simulink model "Proj_v3_wF_Transient"  (R2021b)
settings: Solver=FixedStepAuto  StartTime=0.0  StopTime=10000  FixedStep=10  RelTol=1e-3
values from neighbouring files (symbols this model uses):
  b = 0.0007363716    [Proj_v3_1_mat.m]    (also in Proj_v3_mat.m)
  delta = 3.1e-4    (= 0.00031)    [Proj_v3_1_mat.m]    (also in Proj_v3_mat.m)
  F_L = 0.26    [Proj_v3_1_mat.m]    (also in Proj_v3_mat.m)
  F_P = 0.75    [Proj_v3_1_mat.m]    (also in Proj_v3_mat.m)
  k = 0.7931544    [Proj_v3_1_mat.m]    (also in Proj_v3_mat.m)
  K_m = 16.55418    [Proj_v3_1_mat.m]    (also in Proj_v3_mat.m)
  m = 0.75    [Proj_v3_1_mat.m]    (also in Proj_v3_mat.m)
  r = dose/L    (= 233.333333333)    [Proj_v3_1_mat.m]    (also in Proj_v3_mat.m)
  R_A = 0.0705    [Proj_v3_1_mat.m]    (also in Proj_v3_mat.m)
  S = 0    [Proj_v3_1_mat.m]    (also in Proj_v3_mat.m)
  s = 1.5    [Proj_v3_1_mat.m]    (also in Proj_v3_mat.m)
  V_L = (((W*0.0148)*1000)/rho_liver)/1000    (= 1.17876106195)    [Proj_v3_1_mat.m]    (also in Proj_v3_mat.m)
  V_max = 3.0265    [Proj_v3_1_mat.m]    (also in Proj_v3_mat.m)
  V_T = (W/1.01)*(1-0.064-0.12-0.0148)    (= 71.3940594059)    [Proj_v3_1_mat.m]    (also in Proj_v3_mat.m)
  V_v = 0.064*W    (= 5.76)    [Proj_v3_1_mat.m]    (also in Proj_v3_mat.m)
settings Model: Creator=samil  LastModifiedBy=samil

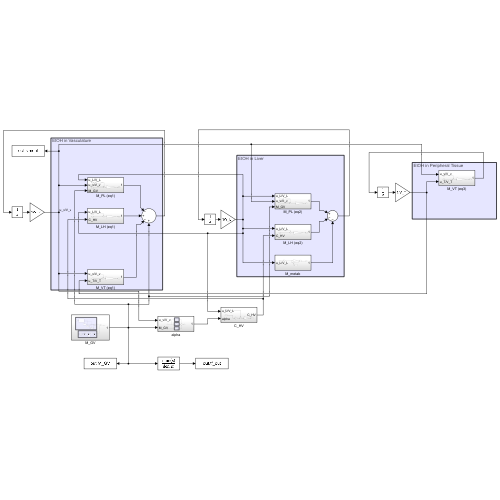
[thumbnail: Simulink's stored preview of the top-level diagram]
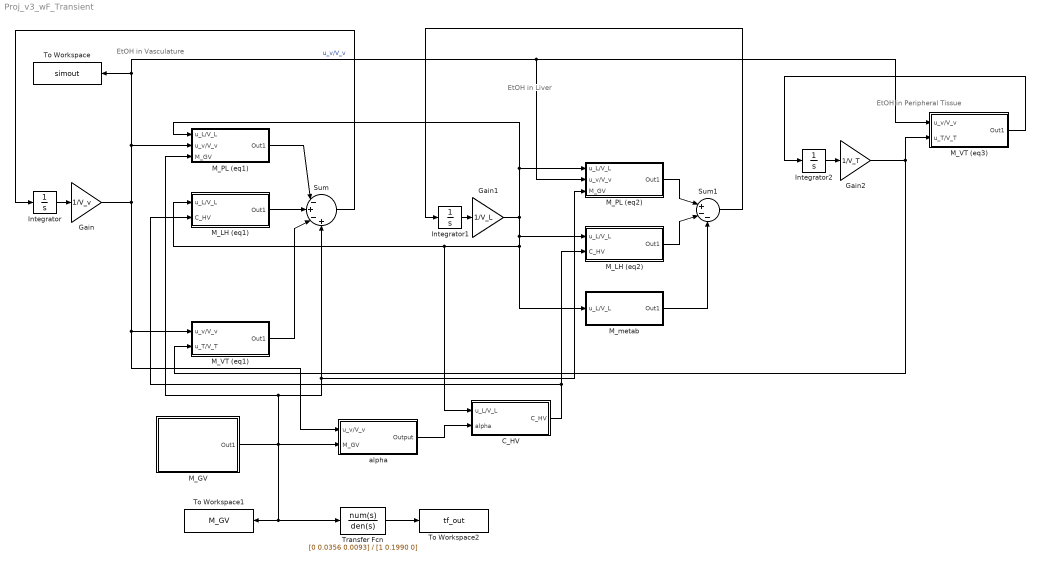
== system Proj_v3_wF_Transient ==
  note: EtOH in Vasculature
  note: EtOH in Peripheral Tissue
  note: EtOH in Liver
  C_HV : Subsystem
  Gain : Gain  Gain=1/V_v
  Gain1 : Gain  Gain=1/V_L
  Gain2 : Gain  Gain=1/V_T
  Integrator : Integrator
  Integrator1 : Integrator
  Integrator2 : Integrator
  M_GV : Subsystem
  M_LH (eq1) : Subsystem
  M_LH (eq2) : Subsystem
  M_PL (eq1) : Subsystem
  M_PL (eq2) : Subsystem
  M_VT (eq1) : Subsystem
  M_VT (eq3) : Subsystem
  M_metab : Subsystem
  Sum : Sum  Inputs=|-+-+
  Sum1 : Sum  Inputs=|+--
  To Workspace : ToWorkspace  VariableName=simout  SaveFormat=Timeseries  SampleTime=-1
  To Workspace1 : ToWorkspace  VariableName=M_GV  SaveFormat=Timeseries  SampleTime=-1
  To Workspace2 : ToWorkspace  VariableName=tf_out  SaveFormat=Timeseries  SampleTime=-1
  Transfer Fcn : TransferFcn  Numerator=[0 0.0356 0.0093]  Denominator=[1 0.1990 0]
  alpha : Subsystem
  wires:
  Integrator1/1 -> Gain1/1
  Integrator2/1 -> Gain2/1
  Integrator/1 -> Gain/1
  Sum/1 -> Integrator/1
  Sum1/1 -> Integrator1/1
  Gain/1 -> To Workspace/1, M_VT (eq3)/1(u_v/V_v), M_PL (eq2)/2(u_v/V_v), M_PL (eq1)/2(u_v/V_v), alpha/1(u_v/V_v), M_VT (eq1)/1(u_v/V_v)  "u_v/V_v"
  C_HV/1(C_HV) -> M_LH (eq1)/2(C_HV), M_LH (eq2)/2(C_HV)
  Gain1/1 -> C_HV/1(u_L/V_L), M_LH (eq1)/1(u_L/V_L), M_metab/1(u_L/V_L), M_LH (eq2)/1(u_L/V_L), M_PL (eq1)/1(u_L/V_L), M_PL (eq2)/1(u_L/V_L)
  Gain2/1 -> M_VT (eq1)/2(u_T/V_T), M_VT (eq3)/2(u_T/V_T)
  alpha/1(Output) -> C_HV/2(alpha)
  M_GV/1(Out1) -> M_PL (eq1)/3(M_GV), Sum/4, M_PL (eq2)/3(M_GV), alpha/2(M_GV), Transfer Fcn/1, To Workspace1/1
  M_PL (eq1)/1(Out1) -> Sum/1
  M_LH (eq1)/1(Out1) -> Sum/2
  M_VT (eq1)/1(Out1) -> Sum/3
  M_PL (eq2)/1(Out1) -> Sum1/1
  M_LH (eq2)/1(Out1) -> Sum1/2
  M_metab/1(Out1) -> Sum1/3
  M_VT (eq3)/1(Out1) -> Integrator2/1
  Transfer Fcn/1 -> To Workspace2/1

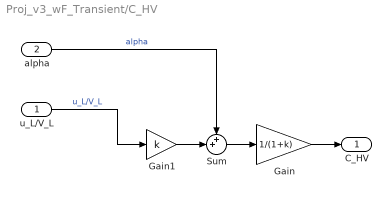
== system Proj_v3_wF_Transient/C_HV ==
  u_L/V_L : Inport
  alpha : Inport  Port=2
  Gain : Gain  Gain=1/(1+k)
  Gain1 : Gain  Gain=k
  Sum : Sum  Inputs=++|
  C_HV : Outport
  wires:
  alpha/1 -> Sum/1  "alpha"
  u_L/V_L/1 -> Gain1/1  "u_L/V_L"
  Gain1/1 -> Sum/2
  Sum/1 -> Gain/1
  Gain/1 -> C_HV/1

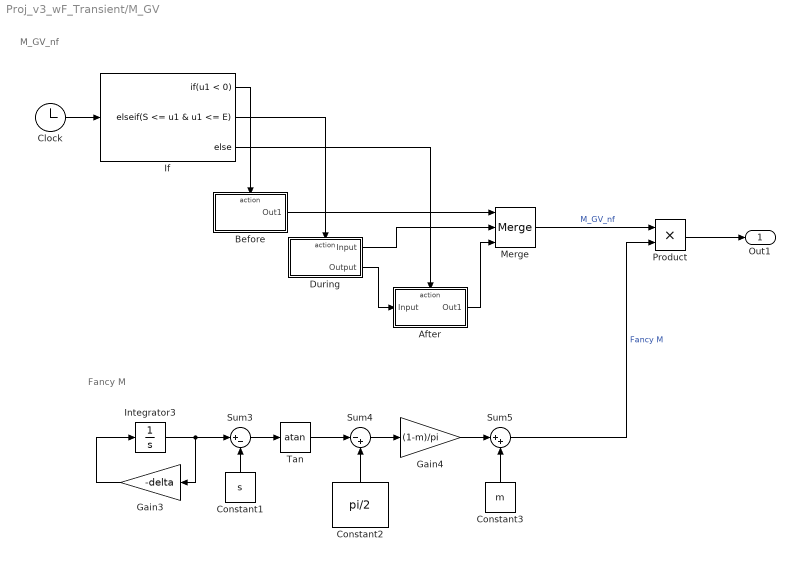
== system Proj_v3_wF_Transient/M_GV ==
  note: Fancy M
  note: M_GV_nf
  After : Subsystem  TreatAsAtomicUnit=on
  Before : Subsystem  TreatAsAtomicUnit=on
  Clock : Clock
  Constant1 : Constant  Value=s
  Constant2 : Constant  Value=pi/2
  Constant3 : Constant  Value=m
  During : Subsystem  TreatAsAtomicUnit=on
  Gain3 : Gain  Gain=-delta
  Gain4 : Gain  Gain=(1-m)/pi
  If : If  IfExpression=u1 < 0  ElseIfExpressions=S <= u1 & u1 <= E
  Integrator3 : Integrator
  Merge : Merge  Inputs=3
  Product : Product
  Sum3 : Sum  Inputs=|+-
  Sum4 : Sum  Inputs=|-+
  Sum5 : Sum  Inputs=|++
  Tan : Trigonometry  Operator=atan
  Out1 : Outport
  wires:
  If/1 -> Before/Action
  If/2 -> During/Action
  Clock/1 -> If/1
  Tan/1 -> Sum4/1
  During/2(Output) -> After/1(Input)
  Product/1 -> Out1/1
  During/1(Input) -> Merge/2
  Integrator3/1 -> Sum3/1, Gain3/1
  If/3 -> After/Action
  Merge/1 -> Product/1  "M_GV_nf"
  Before/1(Out1) -> Merge/1
  Constant3/1 -> Sum5/2
  Sum5/1 -> Product/2  "Fancy M"
  After/1(Out1) -> Merge/3
  Gain4/1 -> Sum5/1
  Sum3/1 -> Tan/1
  Constant1/1 -> Sum3/2
  Constant2/1 -> Sum4/2
  Sum4/1 -> Gain4/1
  Gain3/1 -> Integrator3/1

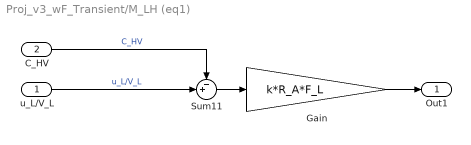
== system Proj_v3_wF_Transient/M_LH (eq1) ==
  u_L/V_L : Inport
  C_HV : Inport  Port=2
  Gain : Gain  Gain=k*R_A*F_L
  Sum11 : Sum  Inputs=-+|
  Out1 : Outport
  wires:
  Sum11/1 -> Gain/1
  u_L/V_L/1 -> Sum11/2  "u_L/V_L"
  C_HV/1 -> Sum11/1  "C_HV"
  Gain/1 -> Out1/1

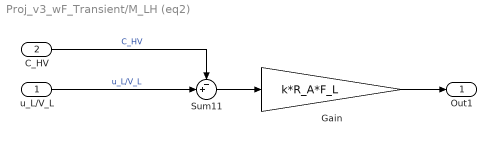
== system Proj_v3_wF_Transient/M_LH (eq2) ==
  u_L/V_L : Inport
  C_HV : Inport  Port=2
  Gain : Gain  Gain=k*R_A*F_L
  Sum11 : Sum  Inputs=-+|
  Out1 : Outport
  wires:
  u_L/V_L/1 -> Sum11/2  "u_L/V_L"
  C_HV/1 -> Sum11/1  "C_HV"
  Sum11/1 -> Gain/1
  Gain/1 -> Out1/1

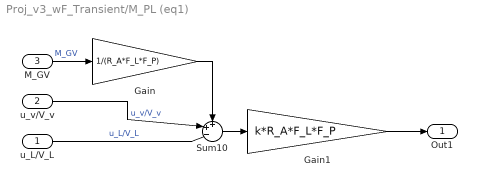
== system Proj_v3_wF_Transient/M_PL (eq1) ==
  u_L/V_L : Inport
  u_v/V_v : Inport  Port=2
  M_GV : Inport  Port=3
  Gain : Gain  Gain=1/(R_A*F_L*F_P)
  Gain1 : Gain  Gain=k*R_A*F_L*F_P
  Sum10 : Sum  Inputs=++-|
  Out1 : Outport
  wires:
  Sum10/1 -> Gain1/1
  u_L/V_L/1 -> Sum10/3  "u_L/V_L"
  u_v/V_v/1 -> Sum10/2  "u_v/V_v"
  M_GV/1 -> Gain/1  "M_GV"
  Gain/1 -> Sum10/1
  Gain1/1 -> Out1/1

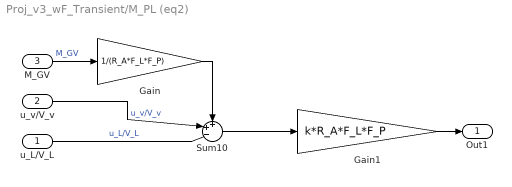
== system Proj_v3_wF_Transient/M_PL (eq2) ==
  u_L/V_L : Inport
  u_v/V_v : Inport  Port=2
  M_GV : Inport  Port=3
  Gain : Gain  Gain=1/(R_A*F_L*F_P)
  Gain1 : Gain  Gain=k*R_A*F_L*F_P
  Sum10 : Sum  Inputs=++-|
  Out1 : Outport
  wires:
  u_L/V_L/1 -> Sum10/3  "u_L/V_L"
  u_v/V_v/1 -> Sum10/2  "u_v/V_v"
  M_GV/1 -> Gain/1  "M_GV"
  Gain/1 -> Sum10/1
  Sum10/1 -> Gain1/1
  Gain1/1 -> Out1/1

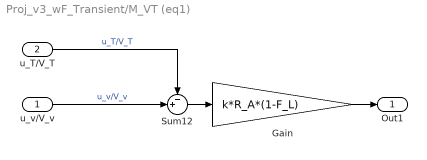
== system Proj_v3_wF_Transient/M_VT (eq1) ==
  u_v/V_v : Inport
  u_T/V_T : Inport  Port=2
  Gain : Gain  Gain=k*R_A*(1-F_L)
  Sum12 : Sum  Inputs=-+|
  Out1 : Outport
  wires:
  Sum12/1 -> Gain/1
  u_v/V_v/1 -> Sum12/2  "u_v/V_v"
  u_T/V_T/1 -> Sum12/1  "u_T/V_T"
  Gain/1 -> Out1/1

== system Proj_v3_wF_Transient/M_VT (eq3) ==
  u_v/V_v : Inport
  u_T/V_T : Inport  Port=2
  Gain : Gain  Gain=k*R_A*(1-F_L)
  Sum12 : Sum  Inputs=-+|
  Out1 : Outport
  wires:
  u_v/V_v/1 -> Sum12/2  "u_v/V_v"
  u_T/V_T/1 -> Sum12/1  "u_T/V_T"
  Sum12/1 -> Gain/1
  Gain/1 -> Out1/1

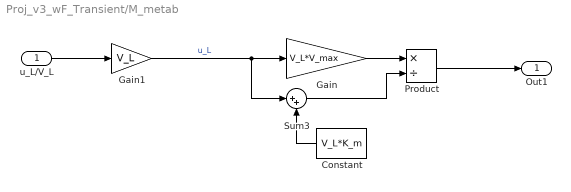
== system Proj_v3_wF_Transient/M_metab ==
  u_L/V_L : Inport
  Constant : Constant  Value=V_L*K_m
  Gain : Gain  Gain=V_L*V_max
  Gain1 : Gain  Gain=V_L
  Product : Product  Inputs=*/
  Sum3 : Sum  Inputs=|++
  Out1 : Outport
  wires:
  Gain/1 -> Product/1
  Constant/1 -> Sum3/2
  Sum3/1 -> Product/2
  Product/1 -> Out1/1
  u_L/V_L/1 -> Gain1/1
  Gain1/1 -> Sum3/1, Gain/1  "u_L"

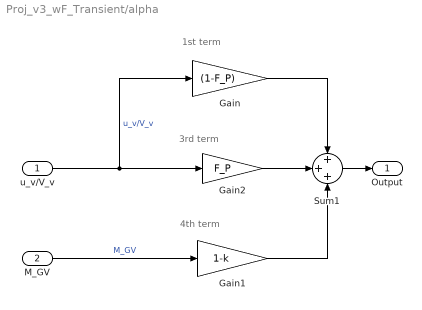
== system Proj_v3_wF_Transient/alpha ==
  note: 4th term
  note: 3rd term
  note: 1st term
  u_v/V_v : Inport
  M_GV : Inport  Port=2
  Gain : Gain  Gain=(1-F_P)
  Gain1 : Gain  Gain=1-k
  Gain2 : Gain  Gain=F_P
  Sum1 : Sum  Inputs=+++
  Output : Outport
  wires:
  u_v/V_v/1 -> Gain/1, Gain2/1  "u_v/V_v"
  M_GV/1 -> Gain1/1  "M_GV"
  Sum1/1 -> Output/1
  Gain2/1 -> Sum1/2
  Gain/1 -> Sum1/1
  Gain1/1 -> Sum1/3

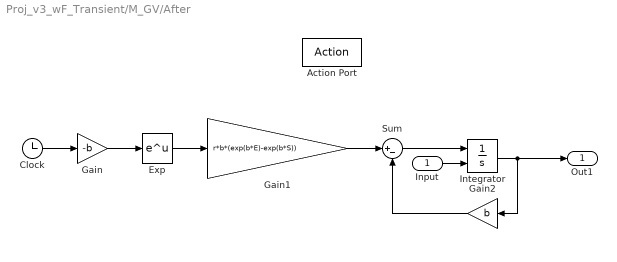
== system Proj_v3_wF_Transient/M_GV/After ==
  Input : Inport
  Action Port : ActionPort  ActionPortLabel=else
  Clock : Clock
  Exp : Math  SaturateOnIntegerOverflow=on
  Gain : Gain  Gain=-b
  Gain1 : Gain  Gain=r*b*(exp(b*E)-exp(b*S))
  Gain2 : Gain  Gain=b
  Integrator : Integrator  InitialConditionSource=external
  Sum : Sum  Inputs=|+-
  Out1 : Outport
  wires:
  Clock/1 -> Gain/1
  Gain/1 -> Exp/1
  Gain1/1 -> Sum/1
  Exp/1 -> Gain1/1
  Sum/1 -> Integrator/1
  Gain2/1 -> Sum/2
  Integrator/1 -> Out1/1, Gain2/1
  Input/1 -> Integrator/2

== system Proj_v3_wF_Transient/M_GV/Before ==
  Action Port : ActionPort  ActionPortLabel=if(u1 < 0)
  Constant : Constant  Value=0
  Out1 : Outport
  wires:
  Constant/1 -> Out1/1

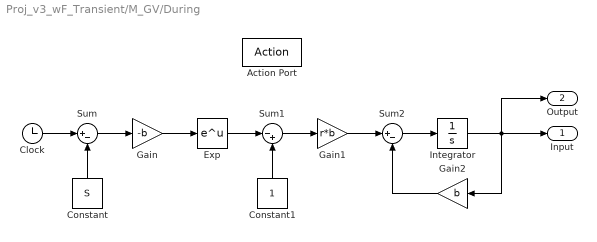
== system Proj_v3_wF_Transient/M_GV/During ==
  Action Port : ActionPort  ActionPortLabel=elseif(S <= u1 & u1 <= E)
  Clock : Clock
  Constant : Constant  Value=S
  Constant1 : Constant
  Exp : Math  SaturateOnIntegerOverflow=on
  Gain : Gain  Gain=-b
  Gain1 : Gain  Gain=r*b
  Gain2 : Gain  Gain=b
  Integrator : Integrator
  Sum : Sum  Inputs=|+-
  Sum1 : Sum  Inputs=|-+
  Sum2 : Sum  Inputs=|+-
  Input : Outport
  Output : Outport  Port=2
  wires:
  Clock/1 -> Sum/1
  Constant/1 -> Sum/2
  Sum/1 -> Gain/1
  Gain/1 -> Exp/1
  Exp/1 -> Sum1/1
  Constant1/1 -> Sum1/2
  Sum1/1 -> Gain1/1
  Gain1/1 -> Sum2/1
  Sum2/1 -> Integrator/1
  Gain2/1 -> Sum2/2
  Integrator/1 -> Output/1, Input/1, Gain2/1
